simulink model "Inner2NoActions"  (Simulink 9.0)
settings: Solver=FixedStepDiscrete  StartTime=0.0  StopTime=20.0  RelTol=1e-3  EnableMultiTasking=on
settings Model: SuppressorTable=22 serialization::archive 11 0 6 0 0 0 0 0  Creator=scaife  LastModifiedBy=ktrinh  ExtModeAutoUpdateStatusClock=off
settings DataIOCC: LimitDataPoints=on  SignalLoggingSaveFormat=ModelDataLogs  SignalLoggingName=sigsOut
settings DebuggingCC: SaveWithParameterizedLinksMsg=none  SignalResolutionControl=TryResolveAllWithWarning  MultiTaskDSMMsg=warning  MultiTaskCondExecSysMsg=none
settings HardwareCC: TargetUnknown=on
settings SFSimCC: SimParseCustomCode=off
settings GRTTargetCC: GeneratePreprocessorConditionals=Disable all  CombineOutputUpdateFcns=off  GRTInterface=on

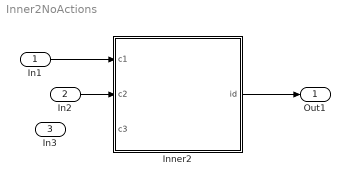
== system Inner2NoActions ==
  In1 : Inport  OutDataTypeStr=boolean
  In2 : Inport  Port=2  OutDataTypeStr=boolean
  In3 : Inport  Port=3  OutDataTypeStr=boolean
  Inner2 : Stateflow chart  TreatAsAtomicUnit=on
  Out1 : Outport
  wires:
  Inner2/1(id) -> Out1/1
  In1/1 -> Inner2/1(c1)
  In2/1 -> Inner2/2(c2)

== stateflow chart Inner2 ==
  state A/
    en: id=1;
    state A1/
      en: id=2;
    state A2/
      en: id=3;
    A -> A [order 1] : [c1]
    A -> A1 [order 2] : [c2]
    A1 -> A : [c3]
    (default) -> A2 : {}
  (default) -> A
  data: c1 input boolean; c2 input boolean; c3 input boolean; id output double
